simulink model "model"  (R2023b)
settings: Solver=VariableStepAuto  StartTime=0  StopTime=10  RelTol=1e-3
settings Model: Creator=Антон  LastModifiedBy=OskolockKoli

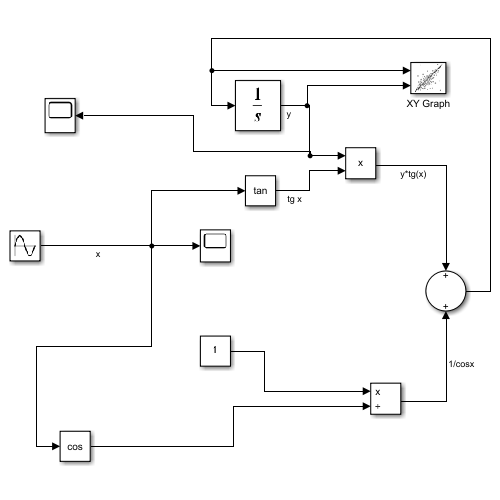
[thumbnail: Simulink's stored preview of the top-level diagram]
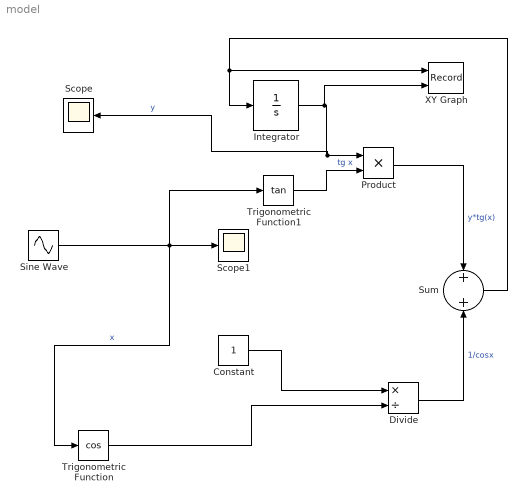
== system model ==
  Constant : Constant
  Divide : Product  Inputs=*/
  Integrator : Integrator  InitialCondition=1
  Product : Product
  Scope : Scope
  Scope1 : Scope
  Sine Wave : Sin  Amplitude=1.5  SampleTime=0
  Sum : Sum  Inputs=+|+
  Trigonometric Function : Trigonometry  Operator=cos
  Trigonometric Function1 : Trigonometry  Operator=tan
  XY Graph : Record  FileSettingsInternal="{\"entries\":[{\"content\":{\"excelSettings\":{\"content\":{},\"type\":\"Streamout.ExcelSettings\"}},\"type\":\"Streamout.FileSettingStorage\",\"uuid\":\"\"}],\"packageUris\":[\"http:\\/\\/schema.mathworks.com\\/mf0\\/streamout_blocks\\/R2020a\"],\"version\":\"1.0\"}"  Layout=[1 1]  SignalsInternal="{\"entries\":[{\"content\":{\"signals\":[{\"content\":{\"blockPath\":[],\"dimensions\":[1],\"domain\":\"\",\"lineColor\":\"#a2142f\",\"plots\":[1],\"port\":1,\"sid\":[\"\"],\"signalID\":173,\"signalName\":\"Sum\"},\"type\":\"RecordBlkView.Signal\",\"uuid\":\"\"},{\"content\":{\"blockPath\":[],\"dimensions\":[1],\"domain\":\"\",\"lineColor\":\"#139fff\",\"plots\":[1],\"port\":2,\"sid\":[\"\"],\"signalID\":177,\"signalName\":\"y\"},\"type\":\"RecordBlkView.Signal\",\"uuid\":\"\"}]},\"type\":\"RecordBlkView.InputSignals\",\"uuid\":\"\"}],\"packageUris\":[\"http:\\/\\/schema.mathworks.com\\/mf0\\/streamout_blocks\\/R2020a\"],\"version\":\"1.0\"}"  VisualizationBindings="{\"xyplotplugin\":{\"info\":[{\"series\":[{\"bindingParametersList\":[{\"parameter\":\"X-Axis\",\"signalID\":173,\"signalName\":\"Sum\"},{\"parameter\":\"Y-Axis\",\"signalID\":177,\"signalName\":\"y\"}],\"seriesID\":13283}],\"subplotID\":1}]}}"  CompatibilityTag=XY
  wires:
  Integrator/1 -> XY Graph/2, Scope/1, Product/1  "y"
  Sine Wave/1 -> Scope1/1, Trigonometric Function/1, Trigonometric Function1/1  "x"
  Trigonometric Function1/1 -> Product/2  "tg x"
  Product/1 -> Sum/1  "y*tg(x)"
  Constant/1 -> Divide/1
  Divide/1 -> Sum/2  "1/cosx"
  Sum/1 -> XY Graph/1, Integrator/1
  Trigonometric Function/1 -> Divide/2
